simulink model "RollOnlySimulation_2010a"  (Simulink 7.5)
settings: Solver=ode45  StartTime=0.0  StopTime=10  RelTol=1e-3
values from neighbouring files (symbols this model uses):
  A_matrix = [0 1;0 0]    [InitSimuLinkModel_basic00.m]
  B_matrix = [0; veh.Ixx]    [InitSimuLinkModel_basic00.m]
undefined symbols (not defined in the file or in its folder): cont, env, sigbuilder_block
settings Model: Creator=admin  LastModifiedBy=admin
settings DebuggingCC: FcnCallInpInsideContextMsg=Enable All
settings GRTTargetCC: CombineOutputUpdateFcns=on

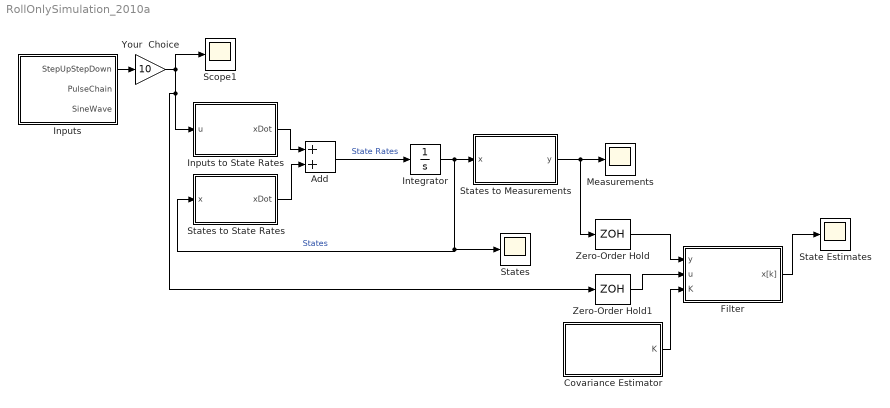
== system RollOnlySimulation_2010a ==
  Add : Sum
  Covariance Estimator : Subsystem
  Filter : Subsystem
  Inputs : Subsystem
  Inputs to State Rates : Subsystem
  Integrator : Integrator  InitialCondition=[0; 0]
  Measurements : Scope
      settings: TimeRange=10  YMin=-2  YMax=10  SaveName=ScopeData2
  Scope1 : Scope
      settings: TimeRange=10  YMin=-10  YMax=10
  State Estimates : Scope
      settings: TimeRange=10  YMin=-0.8  YMax=0.6000000000000001  SaveName=ScopeData3
  States : Scope
      settings: TimeRange=10  YMin=-0.5  YMax=0.5
  States to Measurements : Subsystem
  States to State Rates : Subsystem
  Your  Choice : Gain  Gain=10
  Zero-Order Hold : ZeroOrderHold  SampleTime=cont.LoopPeriod
  Zero-Order Hold1 : ZeroOrderHold  SampleTime=cont.LoopPeriod
  wires:
  Add/1 -> Integrator/1  "State Rates"
  Integrator/1 -> States to Measurements/1(x), States to State Rates/1(x), States/1  "States"
  Inputs to State Rates/1(xDot) -> Add/1
  States to State Rates/1(xDot) -> Add/2
  Inputs/1(StepUpStepDown) -> Your  Choice/1
  States to Measurements/1(y) -> Zero-Order Hold/1, Measurements/1
  Your  Choice/1 -> Scope1/1, Inputs to State Rates/1(u), Zero-Order Hold1/1
  Zero-Order Hold/1 -> Filter/1(y)
  Filter/1(x[k]) -> State Estimates/1
  Covariance Estimator/1(K) -> Filter/3(K)
  Zero-Order Hold1/1 -> Filter/2(u)

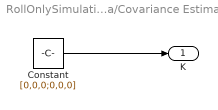
== system RollOnlySimulation_2010a/Covariance Estimator ==
  Constant : Constant  Value=[0,0,0;0,0,0]  SampleTime=cont.LoopPeriod
  K : Outport
  wires:
  Constant/1 -> K/1

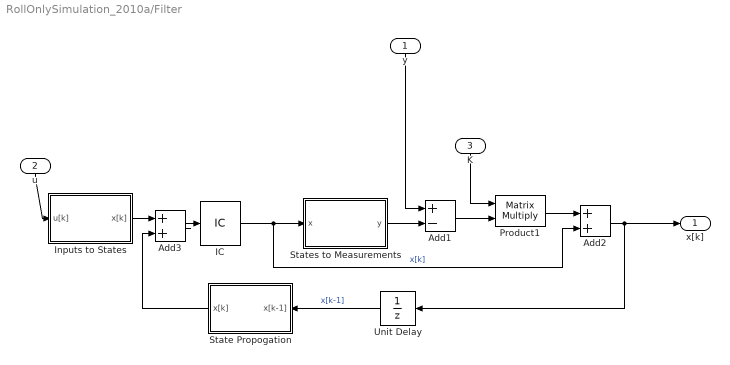
== system RollOnlySimulation_2010a/Filter ==
  y : Inport
  u : Inport  Port=2
  K : Inport  Port=3
  Add1 : Sum  Inputs=+-  SampleTime=cont.LoopPeriod
  Add2 : Sum  SampleTime=cont.LoopPeriod
  Add3 : Sum  SampleTime=cont.LoopPeriod
  IC : InitialCondition  Value=[0 0]  SampleTime=cont.LoopPeriod
  Inputs to States : Subsystem
  Product1 : Product  Multiplication=Matrix(*)  RndMeth=Zero
  State Propogation : Subsystem
  States to Measurements : Subsystem
  Unit Delay : UnitDelay  SampleTime=-1
  x[k] : Outport
  wires:
  IC/1 -> Add2/2, States to Measurements/1(x)  "x[k]"
  Unit Delay/1 -> State Propogation/1(x[k-1])  "x[k-1]"
  Product1/1 -> Add2/1
  y/1 -> Add1/1
  Add1/1 -> Product1/2
  Add2/1 -> x[k]/1, Unit Delay/1
  States to Measurements/1(y) -> Add1/2
  K/1 -> Product1/1
  u/1 -> Inputs to States/1(u[k])
  Inputs to States/1(x[k]) -> Add3/1
  Add3/1 -> IC/1
  State Propogation/1(x[k]) -> Add3/2

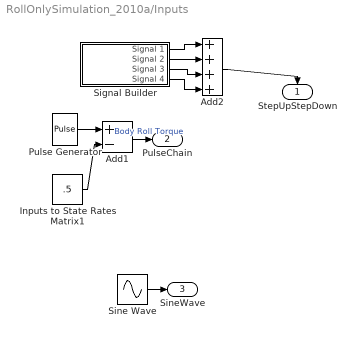
== system RollOnlySimulation_2010a/Inputs ==
  Add1 : Sum  Inputs=+-
  Add2 : Sum  Inputs=++++
  Inputs to State Rates Matrix1 : Constant  Value=.5
  Pulse Generator : DiscretePulseGenerator  PulseType=Time based  Period=10  PulseWidth=50
  Signal Builder : Subsystem  Tag=STV Subsys  LoadFcn=sigbuilder_block('load');  StartFcn=sigbuilder_block('start');  StopFcn=sigbuilder_block('stop');  ClipboardFcn=sigbuilder_block('clipboard');  mask(Sigbuilder block){}
      mask help: Simulink:masks:SigbuilderBlock_MD
      mask init:
      | if ~strcmp(get_param(bdroot(gcbh),'SimulationStatus'),'stopped') tuvar = sigbuilder_block('maskInit'); end
      settings: CopyFcn=sigbuilder_block('copy');  DeleteFcn=sigbuilder_block('delete');  ModelCloseFcn=sigbuilder_block('modelClose');  PreSaveFcn=sigbuilder_block('preSave');  NameChangeFcn=sigbuilder_block('namechange');  OpenFcn=sigbuilder_block('open',[406.5 147 550.5 399.75 ]);  CloseFcn=sigbuilder_block('close');
      mask Display: plot(0,0,100,100,[10,10,40,40,10],[80,20,20,80,80],[40,10],[50,50], [40,27,10],[65,72,56],[40,25,25,10],[28,28,43,43]);
  Sine Wave : Sin  SampleTime=0
  StepUpStepDown : Outport
  PulseChain : Outport  Port=2
  SineWave : Outport  Port=3
  wires:
  Pulse Generator/1 -> Add1/1
  Inputs to State Rates Matrix1/1 -> Add1/2
  Signal Builder/1(Signal 1) -> Add2/1
  Add2/1 -> StepUpStepDown/1
  Sine Wave/1 -> SineWave/1
  Signal Builder/4(Signal 4) -> Add2/4
  Signal Builder/2(Signal 2) -> Add2/2
  Signal Builder/3(Signal 3) -> Add2/3
  Add1/1 -> PulseChain/1  "Body Roll Torque"

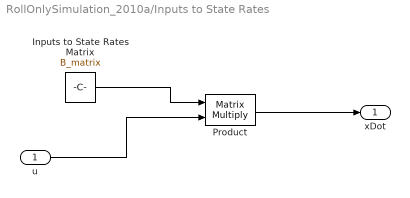
== system RollOnlySimulation_2010a/Inputs to State Rates ==
  u : Inport
  Inputs to State Rates Matrix : Constant  Value=B_matrix
  Product : Product  Multiplication=Matrix(*)  RndMeth=Zero
  xDot : Outport
  wires:
  u/1 -> Product/2
  Product/1 -> xDot/1
  Inputs to State Rates Matrix/1 -> Product/1

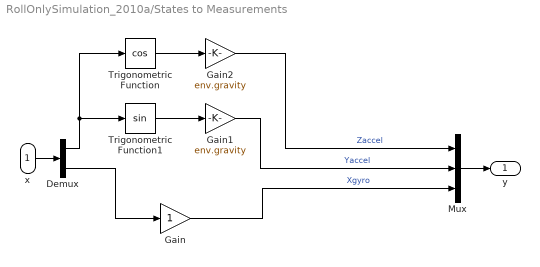
== system RollOnlySimulation_2010a/States to Measurements ==
  x : Inport
  Demux : Demux  Outputs=2
  Gain : Gain
  Gain1 : Gain  Gain=env.gravity
  Gain2 : Gain  Gain=env.gravity
  Mux : Mux  Inputs=3
  Trigonometric Function : Trigonometry  Operator=cos
  Trigonometric Function1 : Trigonometry
  y : Outport
  wires:
  x/1 -> Demux/1
  Demux/2 -> Gain/1
  Demux/1 -> Trigonometric Function1/1, Trigonometric Function/1
  Trigonometric Function1/1 -> Gain1/1
  Trigonometric Function/1 -> Gain2/1
  Mux/1 -> y/1
  Gain2/1 -> Mux/1  "Zaccel"
  Gain1/1 -> Mux/2  "Yaccel"
  Gain/1 -> Mux/3  "Xgyro"

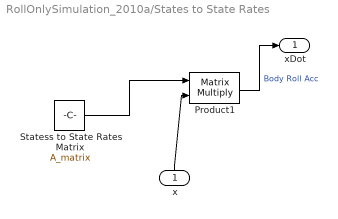
== system RollOnlySimulation_2010a/States to State Rates ==
  x : Inport
  Product1 : Product  Multiplication=Matrix(*)  RndMeth=Zero
  Statess to State Rates Matrix : Constant  Value=A_matrix
  xDot : Outport
  wires:
  Product1/1 -> xDot/1  "Body Roll Acc"
  x/1 -> Product1/2
  Statess to State Rates Matrix/1 -> Product1/1

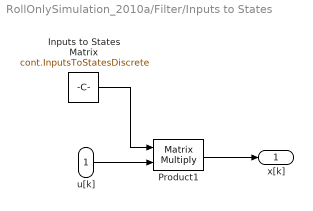
== system RollOnlySimulation_2010a/Filter/Inputs to States ==
  u[k] : Inport
  Inputs to States Matrix : Constant  Value=cont.InputsToStatesDiscrete  SampleTime=cont.LoopPeriod
  Product1 : Product  Multiplication=Matrix(*)  RndMeth=Zero
  x[k] : Outport
  wires:
  u[k]/1 -> Product1/2
  Inputs to States Matrix/1 -> Product1/1
  Product1/1 -> x[k]/1

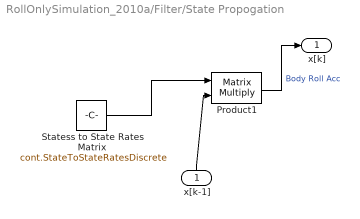
== system RollOnlySimulation_2010a/Filter/State Propogation ==
  x[k-1] : Inport
  Product1 : Product  Multiplication=Matrix(*)  RndMeth=Zero
  Statess to State Rates Matrix : Constant  Value=cont.StateToStateRatesDiscrete  SampleTime=cont.LoopPeriod
  x[k] : Outport
  wires:
  Product1/1 -> x[k]/1  "Body Roll Acc"
  x[k-1]/1 -> Product1/2
  Statess to State Rates Matrix/1 -> Product1/1

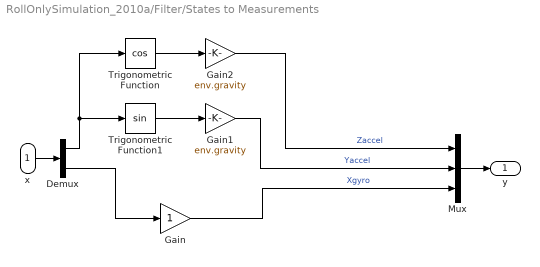
== system RollOnlySimulation_2010a/Filter/States to Measurements ==
  x : Inport
  Demux : Demux  Outputs=2
  Gain : Gain
  Gain1 : Gain  Gain=env.gravity
  Gain2 : Gain  Gain=env.gravity
  Mux : Mux  Inputs=3
  Trigonometric Function : Trigonometry  Operator=cos
  Trigonometric Function1 : Trigonometry
  y : Outport
  wires:
  x/1 -> Demux/1
  Demux/2 -> Gain/1
  Demux/1 -> Trigonometric Function1/1, Trigonometric Function/1
  Trigonometric Function1/1 -> Gain1/1
  Trigonometric Function/1 -> Gain2/1
  Mux/1 -> y/1
  Gain2/1 -> Mux/1  "Zaccel"
  Gain1/1 -> Mux/2  "Yaccel"
  Gain/1 -> Mux/3  "Xgyro"

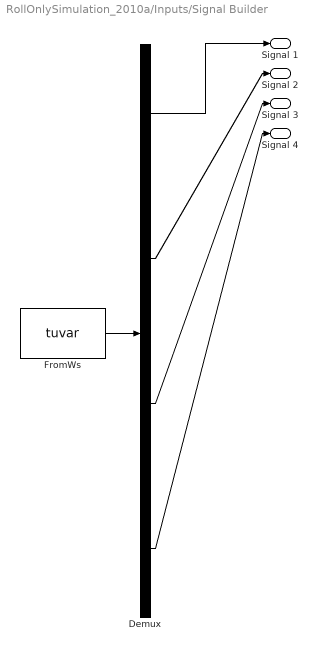
== system RollOnlySimulation_2010a/Inputs/Signal Builder ==
  Demux : Demux  Tag=STV Demux
  FromWs : FromWorkspace  Tag=STV FromWs  VariableName=tuvar  SampleTime=0  SigBuilderData=DataTag0  VnvData=DataTag1
      SigBuilderData=|
      | common.afterFinalStr = 'Extrapolate'
      | common.sampleTime = 0
      | dataSet.timeRange = [0 10]
      | dataSet.name = 'Group 1'
      | sbobj.Groups.Name = 'Group 1'
      | sbobj.Groups.Signals(1).Name = 'Signal 1'
      | sbobj.Groups.Signals(1).XData = [0 1 1 2 2 10]
      | sbobj.Groups.Signals(1).YData = [0 0 1 1 0 0]
      | sbobj.Groups.Signals(2).Name = 'Signal 2'
      | sbobj.Groups.Signals(2).XData = [0 2 2 3 3 10]
      | sbobj.Groups.Signals(2).YData = [0 0 -1 -1 0 0]
      | sbobj.Groups.Signals(3).Name = 'Signal 3'
      | sbobj.Groups.Signals(3).XData = [0 4 4 5 5 10]
      | sbobj.Groups.Signals(3).YData = [0 0 -1 -1 0 0]
      | sbobj.Groups.Signals(4).Name = 'Signal 4'
      | sbobj.Groups.Signals(4).XData = [0 5 5 6 6 10]
      | sbobj.Groups.Signals(4).YData = [0 0 1 1 0 0]
  Signal 1 : Outport  Tag=STV Outport
  Signal 2 : Outport  Tag=STV Outport  Port=2
  Signal 3 : Outport  Tag=STV Outport  Port=3
  Signal 4 : Outport  Tag=STV Outport  Port=4
  wires:
  Demux/1 -> Signal 1/1
  FromWs/1 -> Demux/1
  Demux/2 -> Signal 2/1
  Demux/3 -> Signal 3/1
  Demux/4 -> Signal 4/1
